simulink model "GRM_Airframe"  (R2018b)
settings: Solver=FixedStepAuto  StartTime=0.0  StopTime=T_sim  FixedStep=0.001  RelTol=1e-3
PreLoadFcn:
  | addpath('init_functions');
  | init_grm;
  | addpath('parameters');
  | para_def_grm;
values from neighbouring files (symbols this model uses):
  act_dmp = 0.6322    [para_def_grm.m]
  act_omega = 59.9250    (= 59.925)    [para_def_grm.m]
  aero = load('aero.mat')    [para_def_grm.m]
  c_be = -6.5e-3    (= -0.0065)    [init_grm.m]
  c_h_geop0 = 0    [init_grm.m]
  c_h_geope = 11e3    (= 11000)    [init_grm.m]
  c_pa0 = 101325    [init_grm.m]
  c_pe = -c_g0/c_be/sgc    (= 5.25587981272)    [init_grm.m]
  c_r0 = 6371000.79    [init_grm.m]
  c_rot = 7.292115e-5    (= 7.292115e-05)    [init_grm.m]
  c_Tmp0 = 288.15    [init_grm.m]
  d_siB_0 = 0    [para_def_grm.m]
  d_siB_max = deg2rad(1200)    [para_def_grm.m]
  d_siB_min = deg2rad(-1200)    [para_def_grm.m]
  dd_siB_max = deg2rad(50000)    [para_def_grm.m]
  dd_siB_min = deg2rad(-50000)    [para_def_grm.m]
  de_JBBB_xx = JBBB_xx_0 - JBBB_xx_e    (= 0)    [para_def_grm.m]
  de_JBBB_yy = JBBB_yy_0 - JBBB_yy_e    (= 0)    [para_def_grm.m]
  de_JBBB_zz = JBBB_zz_0 - JBBB_zz_e    (= 0)    [para_def_grm.m]
  de_mM = m_fuel_lookup(end)    [para_def_grm.m]
  F_prp = [450.52;428.7;423.25;391.61;352.34;304.35;266.17;243.26;216.92 ... (first row only)    [para_def_grm.m]
  flag_I_aero_switch = 1    [init_grm.m]
  flag_I_flat = 1    [init_grm.m]
  flag_I_gravity_switch = 1    [init_grm.m]
  flag_I_rot = 0    [init_grm.m]
  hcr = 1.4    [init_grm.m]
  J0PB_e = TBP*J0PP_e*TBP'    [para_def_grm.m]
  JMMM_0 = TBP*J0PP_0*TBP'    [para_def_grm.m]
  JMMM_e = TBP*J0PP_e*TBP'    [para_def_grm.m]
  lat_0 = 0    [init_grm.m]
  lon_0 = 0    [init_grm.m]
  m0 = mB_0    (= 3.30977)    [para_def_grm.m]
  m_fuel_lookup = [0;0.0573;0.1127;0.1667;0.2186;0.2681;0.3149;0.3588 ... (first row only)    [para_def_grm.m]
  mB_0 = 3.30977    [para_def_grm.m]
  mM_0 = 1.119    [para_def_grm.m]
  mM_e = de_mM    [para_def_grm.m]
  p0PB = [x0PB;y0PB;z0PB]    [para_def_grm.m]
  pBII_0 = TIE_0*pBEE_0    [init_grm.m]
  pMPB = [xMPB;yMPB;zMPB]    [para_def_grm.m]
  pNPB = [0;0;0]    [para_def_grm.m]
  qEG_0 = q12_from_T12(TEG)    [init_grm.m]
  qIB_0 = qumul(qIG_0,qGB_0)    [init_grm.m]
  qIE_0 = q12_from_T12(TIE_0)    [init_grm.m]
  sgc = 287.05287    [init_grm.m]
  siB_0 = 0    [para_def_grm.m]
  siB_max = deg2rad(30)    [para_def_grm.m]
  siB_min = deg2rad(-30)    [para_def_grm.m]
  t_prp1 = [0.04;0.28;0.54;1;1.48;1.99;2.51;3;3.5;3.67;3.82;4]    [para_def_grm.m]
  t_prp2 = t_prp2'    [para_def_grm.m]
  Tr3r4 = [1,1,1,1;1,1,-1,-1;-1,1,1,-1]*0.25    [para_def_grm.m]
  tRRR = 0    [para_def_grm.m]
  unc_act_bl = 0    [para_def_grm.m]
  unc_act_off = 0    [para_def_grm.m]
  unc_act_scale = 1    [para_def_grm.m]
  unc_aero_Cl_scale = 1    [para_def_grm.m]
  unc_aero_Cm_scale = 1    [para_def_grm.m]
  unc_aero_Cn_scale = 1    [para_def_grm.m]
  unc_aero_Cx_scale = 1    [para_def_grm.m]
  unc_aero_Cy_scale = 1    [para_def_grm.m]
  unc_aero_Cz_scale = 1    [para_def_grm.m]
  unc_cg_x = 0    [para_def_grm.m]
  unc_cg_y = 0    [para_def_grm.m]
  unc_cg_z = 0    [para_def_grm.m]
  unc_mB_bl = 0    [para_def_grm.m]
  unc_mB_scale = 1    [para_def_grm.m]
  unc_moi_Jxx = 0    [para_def_grm.m]
  unc_moi_Jyy = 0    [para_def_grm.m]
  unc_moi_Jzz = 0    [para_def_grm.m]
  unc_prp_scale = 1    [para_def_grm.m]
  unc_prp_x = 0    [para_def_grm.m]
  unc_prp_y = 0    [para_def_grm.m]
  unc_prp_z = 0    [para_def_grm.m]
  vBII_0 = vBEE_0 + cross(wIEI_0,pBII_0)    [init_grm.m]
  wBIB_0 = r2_from_r1_trans_q21(wBII_0,qBI_0)    [init_grm.m]
  x0PB = -0.5    [para_def_grm.m]
  xMPB = -0.9    [para_def_grm.m]
  y0PB = 0    [para_def_grm.m]
  yMPB = 0    [para_def_grm.m]
  z0PB = 0    [para_def_grm.m]
  zMPB = 0    [para_def_grm.m]
undefined symbols (not defined in the file or in its folder): c_b_WGS, c_flat, c_grav, c_rsma, d_mB_lookup, t_dmB
libraries: simulink_extras x11, simulink x3
(part 3 of 6)

== system GRM_Airframe/GRM_Airframe/aerodynamics/aerodynamic_via_lookup/calc_aero_for_mom/launch_rail ==
  hBE : Inport
  FBAB_c : Inport  Port=2
  Constant1 : Constant  Value=flag_I_aero_switch
  Constant3 : Constant  Value=0
  Subtract : Sum  Inputs=++-
  Switch : Switch  Criteria=u2 > Threshold  Threshold=0.05
  Vector Concatenate : Concatenate  NumInputs=3
  initial_altitude : Subsystem
  FBAB : Outport
  wires:
  initial_altitude/1(hBE_0) -> Subtract/3
  FBAB_c/1 -> Switch/1
  Vector Concatenate/1 -> Switch/3
  Switch/1 -> FBAB/1  "FBAB"
  Constant3/1 -> Vector Concatenate/3, Vector Concatenate/2, Vector Concatenate/1
  Subtract/1 -> Switch/2
  hBE/1 -> Subtract/1
  Constant1/1 -> Subtract/2

== system GRM_Airframe/GRM_Airframe/aerodynamics/aerodynamic_via_lookup/calc_aero_for_mom/launch_rail1 ==
  hBE : Inport
  MBAB_c : Inport  Port=2
  Constant1 : Constant  Value=flag_I_aero_switch
  Constant3 : Constant  Value=0
  Subtract : Sum  Inputs=++-
  Switch : Switch  Criteria=u2 > Threshold  Threshold=0.05
  Vector Concatenate : Concatenate  NumInputs=3
  initial_altitude : Subsystem
  MBAB : Outport
  wires:
  Constant1/1 -> Subtract/2
  hBE/1 -> Subtract/1
  Subtract/1 -> Switch/2
  Constant3/1 -> Vector Concatenate/1, Vector Concatenate/2, Vector Concatenate/3
  Switch/1 -> MBAB/1  "MBAB"
  Vector Concatenate/1 -> Switch/3
  MBAB_c/1 -> Switch/1
  initial_altitude/1(hBE_0) -> Subtract/3

== system GRM_Airframe/GRM_Airframe/aerodynamics/aerodynamic_via_lookup/calc_derivatives/Cl_derivatives_lookup ==
  aero_pre_lookup : Inport
  Bus Creator1 : BusCreator  Inputs=7
  Bus Selector2 : BusSelector  OutputSignals=k_Mach,f_Mach,k_alB,f_alB,k_beB,f_beB
  Cl_Interpolation : Interpolation_n-D  NumberOfTableDimensions=3  Table=aero.Cl  ExtrapMethod=Clip  DiagnosticForOutOfRangeInput=Warning  InternalRulePriority=Speed
      settings: InputPortMap=u0,u1,u2,u3,u4,u5
  Cl_delta_l_Interpolation : Interpolation_n-D  NumberOfTableDimensions=3  Table=aero.Cl_delta_l  ExtrapMethod=Clip  DiagnosticForOutOfRangeInput=Warning  InternalRulePriority=Speed
      settings: InputPortMap=u0,u1,u2,u3,u4,u5
  Cl_delta_m_Interpolation : Interpolation_n-D  NumberOfTableDimensions=3  Table=aero.Cl_delta_m  ExtrapMethod=Clip  DiagnosticForOutOfRangeInput=Warning  InternalRulePriority=Speed
      settings: InputPortMap=u0,u1,u2,u3,u4,u5
  Cl_delta_n_Interpolation : Interpolation_n-D  NumberOfTableDimensions=3  Table=aero.Cl_delta_n  ExtrapMethod=Clip  DiagnosticForOutOfRangeInput=Warning  InternalRulePriority=Speed
      settings: InputPortMap=u0,u1,u2,u3,u4,u5
  Clp_Interpolation : Interpolation_n-D  NumberOfTableDimensions=3  Table=aero.Clp  ExtrapMethod=Clip  DiagnosticForOutOfRangeInput=Warning  InternalRulePriority=Speed
      settings: InputPortMap=u0,u1,u2,u3,u4,u5
  Clq_Interpolation : Interpolation_n-D  NumberOfTableDimensions=3  Table=aero.Clq  ExtrapMethod=Clip  DiagnosticForOutOfRangeInput=Warning  InternalRulePriority=Speed
      settings: InputPortMap=u0,u1,u2,u3,u4,u5
  Clr_Interpolation : Interpolation_n-D  NumberOfTableDimensions=3  Table=aero.Clr  ExtrapMethod=Clip  DiagnosticForOutOfRangeInput=Warning  InternalRulePriority=Speed
      settings: InputPortMap=u0,u1,u2,u3,u4,u5
  Constant : Constant  Value=unc_aero_Cl_scale
  Product : Product
  Cl_deriv : Outport
  wires:
  Product/1 -> Bus Creator1/1  "Cl"
  Constant/1 -> Product/1
  Bus Creator1/1 -> Cl_deriv/1  "Cl_deriv_bus"
  Clp_Interpolation/1 -> Bus Creator1/2  "Clp"
  Cl_delta_l_Interpolation/1 -> Bus Creator1/5  "Cldl"
  aero_pre_lookup/1 -> Bus Selector2/1
  Cl_Interpolation/1 -> Product/2  "Cl"
  Cl_delta_m_Interpolation/1 -> Bus Creator1/6  "Cldm"
  Clr_Interpolation/1 -> Bus Creator1/4  "Clr"
  Clq_Interpolation/1 -> Bus Creator1/3  "Clq"
  Cl_delta_n_Interpolation/1 -> Bus Creator1/7  "Cldn"
  Bus Selector2/5 -> Cl_Interpolation/5, Clp_Interpolation/5, Clq_Interpolation/5, Clr_Interpolation/5, Cl_delta_l_Interpolation/5, Cl_delta_m_Interpolation/5, Cl_delta_n_Interpolation/5  "<k_beB>"
  Bus Selector2/1 -> Cl_Interpolation/1, Clp_Interpolation/1, Clq_Interpolation/1, Clr_Interpolation/1, Cl_delta_l_Interpolation/1, Cl_delta_m_Interpolation/1, Cl_delta_n_Interpolation/1  "<k_Mach>"
  Bus Selector2/2 -> Cl_Interpolation/2, Clp_Interpolation/2, Clq_Interpolation/2, Clr_Interpolation/2, Cl_delta_l_Interpolation/2, Cl_delta_m_Interpolation/2, Cl_delta_n_Interpolation/2  "<f_Mach>"
  Bus Selector2/3 -> Cl_Interpolation/3, Clp_Interpolation/3, Clq_Interpolation/3, Clr_Interpolation/3, Cl_delta_l_Interpolation/3, Cl_delta_m_Interpolation/3, Cl_delta_n_Interpolation/3  "<k_alB>"
  Bus Selector2/4 -> Cl_Interpolation/4, Clp_Interpolation/4, Clq_Interpolation/4, Clr_Interpolation/4, Cl_delta_l_Interpolation/4, Cl_delta_m_Interpolation/4, Cl_delta_n_Interpolation/4  "<f_alB>"
  Bus Selector2/6 -> Cl_Interpolation/6, Clp_Interpolation/6, Clq_Interpolation/6, Clr_Interpolation/6, Cl_delta_l_Interpolation/6, Cl_delta_m_Interpolation/6, Cl_delta_n_Interpolation/6  "<f_beB>"

== system GRM_Airframe/GRM_Airframe/aerodynamics/aerodynamic_via_lookup/calc_derivatives/Cm_derivatives_lookup ==
  aero_pre_lookup : Inport
  Bus Creator1 : BusCreator  Inputs=7
  Bus Selector2 : BusSelector  OutputSignals=k_Mach,f_Mach,k_alB,f_alB,k_beB,f_beB
  Cm_Interpolation : Interpolation_n-D  NumberOfTableDimensions=3  Table=aero.Cm  ExtrapMethod=Clip  DiagnosticForOutOfRangeInput=Warning  InternalRulePriority=Speed
      settings: InputPortMap=u0,u1,u2,u3,u4,u5
  Cm_delta_l_Interpolation : Interpolation_n-D  NumberOfTableDimensions=3  Table=aero.Cm_delta_l  ExtrapMethod=Clip  DiagnosticForOutOfRangeInput=Warning  InternalRulePriority=Speed
      settings: InputPortMap=u0,u1,u2,u3,u4,u5
  Cm_delta_m_Interpolation : Interpolation_n-D  NumberOfTableDimensions=3  Table=aero.Cm_delta_m  ExtrapMethod=Clip  DiagnosticForOutOfRangeInput=Warning  InternalRulePriority=Speed
      settings: InputPortMap=u0,u1,u2,u3,u4,u5
  Cm_delta_n_Interpolation : Interpolation_n-D  NumberOfTableDimensions=3  Table=aero.Cm_delta_n  ExtrapMethod=Clip  DiagnosticForOutOfRangeInput=Warning  InternalRulePriority=Speed
      settings: InputPortMap=u0,u1,u2,u3,u4,u5
  Cmp_Interpolation : Interpolation_n-D  NumberOfTableDimensions=3  Table=aero.Cmp  ExtrapMethod=Clip  DiagnosticForOutOfRangeInput=Warning  InternalRulePriority=Speed
      settings: InputPortMap=u0,u1,u2,u3,u4,u5
  Cmq_Interpolation : Interpolation_n-D  NumberOfTableDimensions=3  Table=aero.Cmq  ExtrapMethod=Clip  DiagnosticForOutOfRangeInput=Warning  InternalRulePriority=Speed
      settings: InputPortMap=u0,u1,u2,u3,u4,u5
  Cmr_Interpolation : Interpolation_n-D  NumberOfTableDimensions=3  Table=aero.Cmr  ExtrapMethod=Clip  DiagnosticForOutOfRangeInput=Warning  InternalRulePriority=Speed
      settings: InputPortMap=u0,u1,u2,u3,u4,u5
  Constant : Constant  Value=unc_aero_Cm_scale
  Product : Product
  Cm_deriv : Outport
  wires:
  Product/1 -> Bus Creator1/1  "Cm"
  Constant/1 -> Product/1
  Bus Selector2/4 -> Cm_Interpolation/4, Cmp_Interpolation/4, Cmq_Interpolation/4, Cmr_Interpolation/4, Cm_delta_l_Interpolation/4, Cm_delta_m_Interpolation/4, Cm_delta_n_Interpolation/4  "<f_alB>"
  Bus Selector2/3 -> Cm_Interpolation/3, Cmp_Interpolation/3, Cmq_Interpolation/3, Cmr_Interpolation/3, Cm_delta_l_Interpolation/3, Cm_delta_m_Interpolation/3, Cm_delta_n_Interpolation/3  "<k_alB>"
  Bus Selector2/2 -> Cm_Interpolation/2, Cmp_Interpolation/2, Cmq_Interpolation/2, Cmr_Interpolation/2, Cm_delta_l_Interpolation/2, Cm_delta_m_Interpolation/2, Cm_delta_n_Interpolation/2  "<f_Mach>"
  Bus Selector2/1 -> Cm_Interpolation/1, Cmp_Interpolation/1, Cmq_Interpolation/1, Cmr_Interpolation/1, Cm_delta_l_Interpolation/1, Cm_delta_m_Interpolation/1, Cm_delta_n_Interpolation/1  "<k_Mach>"
  Bus Selector2/6 -> Cm_Interpolation/6, Cmp_Interpolation/6, Cmq_Interpolation/6, Cmr_Interpolation/6, Cm_delta_l_Interpolation/6, Cm_delta_m_Interpolation/6, Cm_delta_n_Interpolation/6  "<f_beB>"
  aero_pre_lookup/1 -> Bus Selector2/1
  Cmp_Interpolation/1 -> Bus Creator1/2  "Cmp"
  Cm_delta_l_Interpolation/1 -> Bus Creator1/5  "Cmdl"
  Bus Selector2/5 -> Cm_Interpolation/5, Cmp_Interpolation/5, Cmq_Interpolation/5, Cmr_Interpolation/5, Cm_delta_l_Interpolation/5, Cm_delta_m_Interpolation/5, Cm_delta_n_Interpolation/5  "<k_beB>"
  Cmq_Interpolation/1 -> Bus Creator1/3  "Cmq"
  Cm_Interpolation/1 -> Product/2  "Cm"
  Cm_delta_n_Interpolation/1 -> Bus Creator1/7  "Cmdn"
  Cm_delta_m_Interpolation/1 -> Bus Creator1/6  "Cmdm"
  Cmr_Interpolation/1 -> Bus Creator1/4  "Cmr"
  Bus Creator1/1 -> Cm_deriv/1  "Cm_deriv_bus"

== system GRM_Airframe/GRM_Airframe/aerodynamics/aerodynamic_via_lookup/calc_derivatives/Cn_derivatives_lookup ==
  aero_pre_lookup : Inport
  Bus Creator1 : BusCreator  Inputs=7
  Bus Selector1 : BusSelector  OutputSignals=k_Mach,f_Mach,k_alB,f_alB,k_beB,f_beB
  Cn_Interpolation : Interpolation_n-D  NumberOfTableDimensions=3  Table=aero.Cn  ExtrapMethod=Clip  DiagnosticForOutOfRangeInput=Warning  InternalRulePriority=Speed
      settings: InputPortMap=u0,u1,u2,u3,u4,u5
  Cn_delta_l_Interpolation : Interpolation_n-D  NumberOfTableDimensions=3  Table=aero.Cn_delta_l  ExtrapMethod=Clip  DiagnosticForOutOfRangeInput=Warning  InternalRulePriority=Speed
      settings: InputPortMap=u0,u1,u2,u3,u4,u5
  Cn_delta_m_Interpolation : Interpolation_n-D  NumberOfTableDimensions=3  Table=aero.Cn_delta_m  ExtrapMethod=Clip  DiagnosticForOutOfRangeInput=Warning  InternalRulePriority=Speed
      settings: InputPortMap=u0,u1,u2,u3,u4,u5
  Cn_delta_n_Interpolation : Interpolation_n-D  NumberOfTableDimensions=3  Table=aero.Cn_delta_n  ExtrapMethod=Clip  DiagnosticForOutOfRangeInput=Warning  InternalRulePriority=Speed
      settings: InputPortMap=u0,u1,u2,u3,u4,u5
  Cnp_Interpolation : Interpolation_n-D  NumberOfTableDimensions=3  Table=aero.Cnp  ExtrapMethod=Clip  DiagnosticForOutOfRangeInput=Warning  InternalRulePriority=Speed
      settings: InputPortMap=u0,u1,u2,u3,u4,u5
  Cnq_Interpolation : Interpolation_n-D  NumberOfTableDimensions=3  Table=aero.Cnq  ExtrapMethod=Clip  DiagnosticForOutOfRangeInput=Warning  InternalRulePriority=Speed
      settings: InputPortMap=u0,u1,u2,u3,u4,u5
  Cnr_Interpolation : Interpolation_n-D  NumberOfTableDimensions=3  Table=aero.Cnr  ExtrapMethod=Clip  DiagnosticForOutOfRangeInput=Warning  InternalRulePriority=Speed
      settings: InputPortMap=u0,u1,u2,u3,u4,u5
  Constant : Constant  Value=unc_aero_Cn_scale
  Product : Product
  Cn_deriv : Outport
  wires:
  Product/1 -> Bus Creator1/1  "Cn"
  Constant/1 -> Product/1
  Bus Selector1/6 -> Cn_Interpolation/6, Cnp_Interpolation/6, Cnq_Interpolation/6, Cnr_Interpolation/6, Cn_delta_l_Interpolation/6, Cn_delta_m_Interpolation/6, Cn_delta_n_Interpolation/6  "<f_beB>"
  Cn_delta_l_Interpolation/1 -> Bus Creator1/5  "Cndl"
  Cn_delta_n_Interpolation/1 -> Bus Creator1/7  "Cndn"
  Cn_Interpolation/1 -> Product/2  "Cn"
  Cn_delta_m_Interpolation/1 -> Bus Creator1/6  "Cndm"
  Cnq_Interpolation/1 -> Bus Creator1/3  "Cnq"
  Cnr_Interpolation/1 -> Bus Creator1/4  "Cnr"
  Bus Selector1/5 -> Cn_Interpolation/5, Cnp_Interpolation/5, Cnq_Interpolation/5, Cnr_Interpolation/5, Cn_delta_l_Interpolation/5, Cn_delta_m_Interpolation/5, Cn_delta_n_Interpolation/5  "<k_beB>"
  Bus Creator1/1 -> Cn_deriv/1  "Cn_deriv_bus"
  Cnp_Interpolation/1 -> Bus Creator1/2  "Cnp"
  aero_pre_lookup/1 -> Bus Selector1/1
  Bus Selector1/2 -> Cn_Interpolation/2, Cnp_Interpolation/2, Cnq_Interpolation/2, Cnr_Interpolation/2, Cn_delta_l_Interpolation/2, Cn_delta_m_Interpolation/2, Cn_delta_n_Interpolation/2  "<f_Mach>"
  Bus Selector1/1 -> Cn_Interpolation/1, Cnp_Interpolation/1, Cnq_Interpolation/1, Cnr_Interpolation/1, Cn_delta_l_Interpolation/1, Cn_delta_m_Interpolation/1, Cn_delta_n_Interpolation/1  "<k_Mach>"
  Bus Selector1/4 -> Cn_Interpolation/4, Cnp_Interpolation/4, Cnq_Interpolation/4, Cnr_Interpolation/4, Cn_delta_l_Interpolation/4, Cn_delta_m_Interpolation/4, Cn_delta_n_Interpolation/4  "<f_alB>"
  Bus Selector1/3 -> Cn_Interpolation/3, Cnp_Interpolation/3, Cnq_Interpolation/3, Cnr_Interpolation/3, Cn_delta_l_Interpolation/3, Cn_delta_m_Interpolation/3, Cn_delta_n_Interpolation/3  "<k_alB>"

== system GRM_Airframe/GRM_Airframe/aerodynamics/aerodynamic_via_lookup/calc_derivatives/Cx_derivatives_lookup ==
  delta_t : Inport
  hBE : Inport  Port=2
  aero_pre_lookup : Inport  Port=3
  Bus Creator1 : BusCreator  Inputs=10
  Bus Selector1 : BusSelector  OutputSignals=k_Mach,f_Mach,k_alB,f_alB,k_beB,f_beB
  Constant : Constant  Value=unc_aero_Cx_scale
  Cx_Interpolation : Interpolation_n-D  NumberOfTableDimensions=3  Table=aero.Cx  ExtrapMethod=Clip  InternalRulePriority=Speed
      settings: InputPortMap=u0,u1,u2,u3,u4,u5
  Cx_alt_Interpolation : Interpolation_n-D  NumberOfTableDimensions=3  Table=aero.Cx_alt  ExtrapMethod=Clip  InternalRulePriority=Speed
      settings: InputPortMap=u0,u1,u2,u3,u4,u5
  Cx_base_Interpolation : Interpolation_n-D  NumberOfTableDimensions=3  Table=aero.Cx_base  ExtrapMethod=Clip  InternalRulePriority=Speed
      settings: InputPortMap=u0,u1,u2,u3,u4,u5
  Cx_delta_l_Interpolation : Interpolation_n-D  NumberOfTableDimensions=3  Table=aero.Cx_delta_l  ExtrapMethod=Clip  InternalRulePriority=Speed
      settings: InputPortMap=u0,u1,u2,u3,u4,u5
  Cx_delta_m_Interpolation : Interpolation_n-D  NumberOfTableDimensions=3  Table=aero.Cx_delta_m  ExtrapMethod=Clip  InternalRulePriority=Speed
      settings: InputPortMap=u0,u1,u2,u3,u4,u5
  Cx_delta_n_Interpolation : Interpolation_n-D  NumberOfTableDimensions=3  Table=aero.Cx_delta_n  ExtrapMethod=Clip  InternalRulePriority=Speed
      settings: InputPortMap=u0,u1,u2,u3,u4,u5
  Cx_delta_t_Interpolation : Interpolation_n-D  NumberOfTableDimensions=3  Table=aero.Cx_delta_t  ExtrapMethod=Clip  InternalRulePriority=Speed
      settings: InputPortMap=u0,u1,u2,u3,u4,u5
  Cxp_Interpolation : Interpolation_n-D  NumberOfTableDimensions=3  Table=aero.Cxp  ExtrapMethod=Clip  InternalRulePriority=Speed
      settings: InputPortMap=u0,u1,u2,u3,u4,u5
  Cxq_Interpolation : Interpolation_n-D  NumberOfTableDimensions=3  Table=aero.Cxq  ExtrapMethod=Clip  InternalRulePriority=Speed
      settings: InputPortMap=u0,u1,u2,u3,u4,u5
  Cxr_Interpolation : Interpolation_n-D  NumberOfTableDimensions=3  Table=aero.Cxr  ExtrapMethod=Clip  InternalRulePriority=Speed
      settings: InputPortMap=u0,u1,u2,u3,u4,u5
  Prelookup_altitude : PreLookup  BreakpointsData=aero.hoehe
  Prelookup_delta_t : PreLookup  BreakpointsData=aero.delta_t
  Product : Product
  Cx_deriv : Outport
  wires:
  Constant/1 -> Product/1
  Product/1 -> Bus Creator1/1  "Cx"
  Cx_delta_n_Interpolation/1 -> Bus Creator1/7  "Cxdn"
  Cx_delta_m_Interpolation/1 -> Bus Creator1/6  "Cxdm"
  Cx_delta_l_Interpolation/1 -> Bus Creator1/5  "Cxdl"
  delta_t/1 -> Prelookup_delta_t/1
  Bus Creator1/1 -> Cx_deriv/1  "Cx_deriv_bus"
  Prelookup_altitude/2 -> Cx_alt_Interpolation/6
  Prelookup_altitude/1 -> Cx_alt_Interpolation/5
  hBE/1 -> Prelookup_altitude/1
  aero_pre_lookup/1 -> Bus Selector1/1
  Prelookup_delta_t/1 -> Cx_delta_t_Interpolation/5
  Bus Selector1/1 -> Cx_Interpolation/1, Cxp_Interpolation/1, Cxq_Interpolation/1, Cxr_Interpolation/1, Cx_delta_l_Interpolation/1, Cx_alt_Interpolation/1, Cx_delta_t_Interpolation/1, Cx_base_Interpolation/1, Cx_delta_n_Interpolation/1, Cx_delta_m_Interpolation/1  "<k_Mach>"
  Bus Selector1/2 -> Cx_Interpolation/2, Cxp_Interpolation/2, Cxq_Interpolation/2, Cxr_Interpolation/2, Cx_delta_l_Interpolation/2, Cx_base_Interpolation/2, Cx_alt_Interpolation/2, Cx_delta_t_Interpolation/2, Cx_delta_n_Interpolation/2, Cx_delta_m_Interpolation/2  "<f_Mach>"
  Prelookup_delta_t/2 -> Cx_delta_t_Interpolation/6
  Bus Selector1/3 -> Cx_Interpolation/3, Cxp_Interpolation/3, Cxq_Interpolation/3, Cxr_Interpolation/3, Cx_delta_l_Interpolation/3, Cx_alt_Interpolation/3, Cx_delta_t_Interpolation/3, Cx_base_Interpolation/3, Cx_delta_n_Interpolation/3, Cx_delta_m_Interpolation/3  "<k_alB>"
  Bus Selector1/6 -> Cxp_Interpolation/6, Cxq_Interpolation/6, Cxr_Interpolation/6, Cx_delta_l_Interpolation/6, Cx_base_Interpolation/6, Cx_delta_n_Interpolation/6, Cx_delta_m_Interpolation/6, Cx_Interpolation/6  "<f_beB>"
  Bus Selector1/4 -> Cx_Interpolation/4, Cxp_Interpolation/4, Cxq_Interpolation/4, Cxr_Interpolation/4, Cx_delta_l_Interpolation/4, Cx_alt_Interpolation/4, Cx_delta_t_Interpolation/4, Cx_base_Interpolation/4, Cx_delta_n_Interpolation/4, Cx_delta_m_Interpolation/4  "<f_alB>"
  Cxp_Interpolation/1 -> Bus Creator1/2  "Cxp"
  Cx_delta_t_Interpolation/1 -> Bus Creator1/10  "Cx_alB_t"
  Cxr_Interpolation/1 -> Bus Creator1/4  "Cxr"
  Cxq_Interpolation/1 -> Bus Creator1/3  "Cxq"
  Cx_base_Interpolation/1 -> Bus Creator1/8  "Cx_base"
  Cx_Interpolation/1 -> Product/2  "Cx"
  Cx_alt_Interpolation/1 -> Bus Creator1/9  "Cx_alt"
  Bus Selector1/5 -> Cxp_Interpolation/5, Cxq_Interpolation/5, Cxr_Interpolation/5, Cx_delta_l_Interpolation/5, Cx_base_Interpolation/5, Cx_delta_n_Interpolation/5, Cx_delta_m_Interpolation/5, Cx_Interpolation/5  "<k_beB>"

== system GRM_Airframe/GRM_Airframe/aerodynamics/aerodynamic_via_lookup/calc_derivatives/Cy_derivatives_lookup ==
  aero_pre_lookup : Inport
  Bus Creator1 : BusCreator  Inputs=7
  Bus Selector1 : BusSelector  OutputSignals=k_Mach,f_Mach,k_alB,f_alB,k_beB,f_beB
  Constant : Constant  Value=unc_aero_Cy_scale
  Cy_Interpolation : Interpolation_n-D  NumberOfTableDimensions=3  Table=aero.Cy  ExtrapMethod=Clip  InternalRulePriority=Speed
      settings: InputPortMap=u0,u1,u2,u3,u4,u5
  Cy_delta_l_Interpolation : Interpolation_n-D  NumberOfTableDimensions=3  Table=aero.Cy_delta_l  ExtrapMethod=Clip  InternalRulePriority=Speed
      settings: InputPortMap=u0,u1,u2,u3,u4,u5
  Cy_delta_m_Interpolation : Interpolation_n-D  NumberOfTableDimensions=3  Table=aero.Cy_delta_m  ExtrapMethod=Clip  InternalRulePriority=Speed
      settings: InputPortMap=u0,u1,u2,u3,u4,u5
  Cy_delta_n_Interpolation : Interpolation_n-D  NumberOfTableDimensions=3  Table=aero.Cy_delta_n  ExtrapMethod=Clip  InternalRulePriority=Speed
      settings: InputPortMap=u0,u1,u2,u3,u4,u5
  Cyp_Interpolation : Interpolation_n-D  NumberOfTableDimensions=3  Table=aero.Cyp  ExtrapMethod=Clip  InternalRulePriority=Speed
      settings: InputPortMap=u0,u1,u2,u3,u4,u5
  Cyq_Interpolation : Interpolation_n-D  NumberOfTableDimensions=3  Table=aero.Cyq  ExtrapMethod=Clip  InternalRulePriority=Speed
      settings: InputPortMap=u0,u1,u2,u3,u4,u5
  Cyr_Interpolation : Interpolation_n-D  NumberOfTableDimensions=3  Table=aero.Cyr  ExtrapMethod=Clip  InternalRulePriority=Speed
      settings: InputPortMap=u0,u1,u2,u3,u4,u5
  Product : Product
  Cy_deriv : Outport
  wires:
  Product/1 -> Bus Creator1/1  "Cy"
  Constant/1 -> Product/1
  Cyq_Interpolation/1 -> Bus Creator1/3  "Cyq"
  Cyr_Interpolation/1 -> Bus Creator1/4  "Cyr"
  Bus Creator1/1 -> Cy_deriv/1  "Cy_deriv_bus"
  Cy_delta_m_Interpolation/1 -> Bus Creator1/6  "Cydm"
  Cy_delta_l_Interpolation/1 -> Bus Creator1/5  "Cydl"
  Cyp_Interpolation/1 -> Bus Creator1/2  "Cyp"
  aero_pre_lookup/1 -> Bus Selector1/1
  Bus Selector1/2 -> Cy_Interpolation/2, Cyp_Interpolation/2, Cyq_Interpolation/2, Cyr_Interpolation/2, Cy_delta_l_Interpolation/2, Cy_delta_m_Interpolation/2, Cy_delta_n_Interpolation/2  "<f_Mach>"
  Bus Selector1/1 -> Cy_Interpolation/1, Cyp_Interpolation/1, Cyq_Interpolation/1, Cyr_Interpolation/1, Cy_delta_l_Interpolation/1, Cy_delta_m_Interpolation/1, Cy_delta_n_Interpolation/1  "<k_Mach>"
  Bus Selector1/3 -> Cy_Interpolation/3, Cyp_Interpolation/3, Cyq_Interpolation/3, Cyr_Interpolation/3, Cy_delta_l_Interpolation/3, Cy_delta_m_Interpolation/3, Cy_delta_n_Interpolation/3  "<k_alB>"
  Bus Selector1/4 -> Cy_Interpolation/4, Cyp_Interpolation/4, Cyq_Interpolation/4, Cyr_Interpolation/4, Cy_delta_l_Interpolation/4, Cy_delta_m_Interpolation/4, Cy_delta_n_Interpolation/4  "<f_alB>"
  Bus Selector1/6 -> Cy_Interpolation/6, Cyp_Interpolation/6, Cyq_Interpolation/6, Cyr_Interpolation/6, Cy_delta_l_Interpolation/6, Cy_delta_m_Interpolation/6, Cy_delta_n_Interpolation/6  "<f_beB>"
  Bus Selector1/5 -> Cy_Interpolation/5, Cyp_Interpolation/5, Cyq_Interpolation/5, Cyr_Interpolation/5, Cy_delta_l_Interpolation/5, Cy_delta_m_Interpolation/5, Cy_delta_n_Interpolation/5  "<k_beB>"
  Cy_delta_n_Interpolation/1 -> Bus Creator1/7  "Cydn"
  Cy_Interpolation/1 -> Product/2  "Cy"

== system GRM_Airframe/GRM_Airframe/aerodynamics/aerodynamic_via_lookup/calc_derivatives/Cz_derivatives_lookup ==
  aero_pre_lookup : Inport
  Bus Creator1 : BusCreator  Inputs=7
  Bus Selector2 : BusSelector  OutputSignals=k_Mach,f_Mach,k_alB,f_alB,k_beB,f_beB
  Constant : Constant  Value=unc_aero_Cz_scale
  Cz_Interpolation : Interpolation_n-D  NumberOfTableDimensions=3  Table=aero.Cz  ExtrapMethod=Clip  DiagnosticForOutOfRangeInput=Warning  InternalRulePriority=Speed
      settings: InputPortMap=u0,u1,u2,u3,u4,u5
  Cz_delta_l_Interpolation : Interpolation_n-D  NumberOfTableDimensions=3  Table=aero.Cz_delta_l  ExtrapMethod=Clip  DiagnosticForOutOfRangeInput=Warning  InternalRulePriority=Speed
      settings: InputPortMap=u0,u1,u2,u3,u4,u5
  Cz_delta_m_Interpolation : Interpolation_n-D  NumberOfTableDimensions=3  Table=aero.Cz_delta_m  ExtrapMethod=Clip  DiagnosticForOutOfRangeInput=Warning  InternalRulePriority=Speed
      settings: InputPortMap=u0,u1,u2,u3,u4,u5
  Cz_delta_n_Interpolation : Interpolation_n-D  NumberOfTableDimensions=3  Table=aero.Cz_delta_n  ExtrapMethod=Clip  DiagnosticForOutOfRangeInput=Warning  InternalRulePriority=Speed
      settings: InputPortMap=u0,u1,u2,u3,u4,u5
  Czp_Interpolation : Interpolation_n-D  NumberOfTableDimensions=3  Table=aero.Czp  ExtrapMethod=Clip  DiagnosticForOutOfRangeInput=Warning  InternalRulePriority=Speed
      settings: InputPortMap=u0,u1,u2,u3,u4,u5
  Czq_Interpolation : Interpolation_n-D  NumberOfTableDimensions=3  Table=aero.Czq  ExtrapMethod=Clip  DiagnosticForOutOfRangeInput=Warning  InternalRulePriority=Speed
      settings: InputPortMap=u0,u1,u2,u3,u4,u5
  Czr_Interpolation : Interpolation_n-D  NumberOfTableDimensions=3  Table=aero.Czr  ExtrapMethod=Clip  DiagnosticForOutOfRangeInput=Warning  InternalRulePriority=Speed
      settings: InputPortMap=u0,u1,u2,u3,u4,u5
  Product : Product
  Cz_deriv : Outport
  wires:
  Product/1 -> Bus Creator1/1  "Cz"
  Constant/1 -> Product/1
  Czr_Interpolation/1 -> Bus Creator1/4  "Czr"
  Czp_Interpolation/1 -> Bus Creator1/2  "Czp"
  aero_pre_lookup/1 -> Bus Selector2/1
  Czq_Interpolation/1 -> Bus Creator1/3  "Czq"
  Bus Creator1/1 -> Cz_deriv/1  "Cz_deriv_bus"
  Cz_delta_l_Interpolation/1 -> Bus Creator1/5  "Czdl"
  Cz_delta_n_Interpolation/1 -> Bus Creator1/7  "Czdn"
  Bus Selector2/3 -> Cz_Interpolation/3, Czp_Interpolation/3, Czq_Interpolation/3, Czr_Interpolation/3, Cz_delta_l_Interpolation/3, Cz_delta_m_Interpolation/3, Cz_delta_n_Interpolation/3  "<k_alB>"
  Bus Selector2/6 -> Cz_Interpolation/6, Czp_Interpolation/6, Czq_Interpolation/6, Czr_Interpolation/6, Cz_delta_l_Interpolation/6, Cz_delta_m_Interpolation/6, Cz_delta_n_Interpolation/6  "<f_beB>"
  Cz_delta_m_Interpolation/1 -> Bus Creator1/6  "Czdm"
  Cz_Interpolation/1 -> Product/2  "Cz"
  Bus Selector2/5 -> Cz_Interpolation/5, Czp_Interpolation/5, Czq_Interpolation/5, Czr_Interpolation/5, Cz_delta_l_Interpolation/5, Cz_delta_m_Interpolation/5, Cz_delta_n_Interpolation/5  "<k_beB>"
  Bus Selector2/1 -> Cz_Interpolation/1, Czp_Interpolation/1, Czq_Interpolation/1, Czr_Interpolation/1, Cz_delta_l_Interpolation/1, Cz_delta_m_Interpolation/1, Cz_delta_n_Interpolation/1  "<k_Mach>"
  Bus Selector2/2 -> Cz_Interpolation/2, Czp_Interpolation/2, Czq_Interpolation/2, Czr_Interpolation/2, Cz_delta_l_Interpolation/2, Cz_delta_m_Interpolation/2, Cz_delta_n_Interpolation/2  "<f_Mach>"
  Bus Selector2/4 -> Cz_Interpolation/4, Czp_Interpolation/4, Czq_Interpolation/4, Czr_Interpolation/4, Cz_delta_l_Interpolation/4, Cz_delta_m_Interpolation/4, Cz_delta_n_Interpolation/4  "<f_alB>"

== system GRM_Airframe/GRM_Airframe/aerodynamics/aerodynamic_via_lookup/calc_derivatives/aerodynamics_pre_lookup ==
  alB : Inport
  beB : Inport  Port=2
  Ma : Inport  Port=3
  Bus Creator1 : BusCreator  Inputs=6
  Prelookup_Mach : PreLookup  BreakpointsData=aero.Ma
  Prelookup_alB : PreLookup  BreakpointsData=aero.alpha
  Prelookup_beB : PreLookup  BreakpointsData=aero.beta
  aero_pre_lookup : Outport
  wires:
  beB/1 -> Prelookup_beB/1
  alB/1 -> Prelookup_alB/1
  Prelookup_beB/2 -> Bus Creator1/6  "f_beB"
  Prelookup_beB/1 -> Bus Creator1/5  "k_beB"
  Prelookup_Mach/1 -> Bus Creator1/1  "k_Mach"
  Prelookup_Mach/2 -> Bus Creator1/2  "f_Mach"
  Ma/1 -> Prelookup_Mach/1
  Prelookup_alB/2 -> Bus Creator1/4  "f_alB"
  Prelookup_alB/1 -> Bus Creator1/3  "k_alB"
  Bus Creator1/1 -> aero_pre_lookup/1  "aero_pre_lookup_bus"

== system GRM_Airframe/GRM_Airframe/aerodynamics/aerodynamic_via_lookup/calc_derivatives/calc_total_deflection_angle ==
  etB_deg : Inport
  zeB_deg : Inport  Port=2
  alB : Inport  Port=3
  beB : Inport  Port=4
  Abs : Abs
  Abs1 : Abs
  Abs2 : Abs
  Add : Sum
  Constant3 : Constant  Value=2
  Degrees to Radians : simulink_extras/Transformations/Degrees to Radians
  Degrees to Radians1 : simulink_extras/Transformations/Degrees to Radians
  Divide2 : Product  Inputs=**/
  Product1 : Product
  Product6 : Product
  Product7 : Product
  Radians to Degrees1 : simulink_extras/Transformations/Radians to Degrees
  Saturation : Saturate  UpperLimit=inf  LowerLimit=100*eps
      settings: AttributesFormatString=|
      | %<UpperLimit>
      | %<LowerLimit>
  Sqrt : Sqrt  SaturateOnIntegerOverflow=on
  Trigonometric Function : Trigonometry  Operator=acos
  Trigonometric Function1 : Trigonometry  Operator=cos
  Trigonometric Function2 : Trigonometry  Operator=cos
  delta_t : Outport
  wires:
  Radians to Degrees1/1 -> Saturation/1  "alB_t_deg"
  Trigonometric Function/1 -> Radians to Degrees1/1  "alB_t"
  Degrees to Radians1/1 -> Trigonometric Function2/1
  Degrees to Radians/1 -> Trigonometric Function1/1
  Abs2/1 -> delta_t/1  "delta_t"
  alB/1 -> Degrees to Radians/1, Abs/1
  Product1/1 -> Trigonometric Function/1
  Sqrt/1 -> Divide2/2
  Product7/1 -> Add/2
  beB/1 -> Degrees to Radians1/1, Abs1/1
  Add/1 -> Divide2/1
  Trigonometric Function1/1 -> Product1/1
  Constant3/1 -> Sqrt/1
  zeB_deg/1 -> Product7/2
  Abs/1 -> Product6/1
  etB_deg/1 -> Product6/2
  Trigonometric Function2/1 -> Product1/2
  Divide2/1 -> Abs2/1
  Abs1/1 -> Product7/1
  Saturation/1 -> Divide2/3
  Product6/1 -> Add/1

== system GRM_Airframe/GRM_Airframe/environment/WGS84_Gravitation/WGS84_2_ECEF/WGS84 Transformation Parameter  ==
  phi : Inport
  Add2 : Sum  Inputs=+-
  Divide : Product  Inputs=**
  Divide1 : Product  Inputs=**
  Divide2 : Product  Inputs=**
  Divide3 : Product  Inputs=/*
  Sqrt : Sqrt  SaturateOnIntegerOverflow=on
  Subsystem : Subsystem
  Trigonometric Function : Trigonometry
  "WGS84 Semi-major Axis, [m]" : Constant  Value=c_rsma
  "WGS84 Semi-minor Axis, [m]" : Constant  Value=c_b_WGS
  a3 : Constant
  N : Outport
  e : Outport  Port=2
  wires:
  phi/1 -> Trigonometric Function/1
  Add2/1 -> Sqrt/1
  Subsystem/1(e) -> Divide/1, Divide/2, e/1
  Divide/1 -> Divide2/2  "e^2"
  Trigonometric Function/1 -> Divide1/1, Divide1/2
  Divide2/1 -> Add2/2
  a3/1 -> Add2/1
  Sqrt/1 -> Divide3/1
  Divide3/1 -> N/1  "N"
  Divide1/1 -> Divide2/1  "sin(phi)^2"
  "WGS84 Semi-major Axis, [m]"/1 -> Divide3/2, Subsystem/2(a)  "c_rsma"
  "WGS84 Semi-minor Axis, [m]"/1 -> Subsystem/1(b)  "c_b_WGS"

== system GRM_Airframe/GRM_Airframe/environment/atmosphere_static_ISO_2533/tmp_and_pressure_ISO_2533/static_Temperature ==
  Tmp_ref : Inport
  h_geop : Inport  Port=2
  h_geop_ref : Inport  Port=3
  Add : Sum
  Product : Product
  Subtract : Sum  Inputs=+-
  Tmp_gradient_tropo : Constant  Value=c_be
  Tmp : Outport
  wires:
  h_geop_ref/1 -> Subtract/2
  h_geop/1 -> Subtract/1
  Tmp_ref/1 -> Add/1
  Add/1 -> Tmp/1  "Tmp"
  Product/1 -> Add/2
  Tmp_gradient_tropo/1 -> Product/1
  Subtract/1 -> Product/2

== system GRM_Airframe/GRM_Airframe/environment/atmosphere_static_ISO_2533/tmp_and_pressure_ISO_2533/static_pressure ==
  h_geop_ref : Inport
  h_geop : Inport  Port=2
  Tmp_ref : Inport  Port=3
  pa_ref : Inport  Port=4
  Add : Sum
  Constant1 : Constant
  Divide : Product  Inputs=*/*
  Math Function : Math  Operator=pow  SaturateOnIntegerOverflow=on
  Product : Product
  Subtract : Sum  Inputs=-+
  Tmp_gradient_tropo : Constant  Value=c_be
  pressure_exponent : Constant  Value=c_pe
  pa : Outport
  wires:
  Tmp_gradient_tropo/1 -> Divide/3
  Product/1 -> pa/1  "pa"
  Constant1/1 -> Add/1
  Subtract/1 -> Divide/1
  Math Function/1 -> Product/1
  pa_ref/1 -> Product/2
  Add/1 -> Math Function/1
  Tmp_ref/1 -> Divide/2
  h_geop_ref/1 -> Subtract/1
  Divide/1 -> Add/2
  h_geop/1 -> Subtract/2
  pressure_exponent/1 -> Math Function/2

== system GRM_Airframe/GRM_Airframe/gravity/launch_rail/initial_altitude/trafo_E_to_geodetic ==
  note: Inputs [size]:
      |
      | position_E [3]
  note: Outputs [size]:
      |
      | geodetic longitude [1]
      | geodetic latitude [1]
      | geodetic altitude [1]
  pBEE : Inport
  Geodetic_altitude : Subsystem
  Geodetic_latitude : Subsystem
  Selector1 : Selector  IndexMode=Zero-based  InputPortWidth=3  IndexOptions=Index vector (dialog)  Indices=1  OutputSizes=1
  Selector2 : Selector  IndexMode=Zero-based  InputPortWidth=3  IndexOptions=Index vector (dialog)  Indices=0  OutputSizes=1
  Trigonometric Function1 : Trigonometry  Operator=atan2
  c_flat : Constant  Value=c_flat
  c_rsma : Constant  Value=c_rsma
  lon : Outport
  lat : Outport  Port=2
  alt : Outport  Port=3
  wires:
  pBEE/1 -> Geodetic_altitude/1(pBEE), Geodetic_latitude/1(pBEE), Selector2/1, Selector1/1  "pBEE"
  Trigonometric Function1/1 -> lon/1  "lon"
  Geodetic_altitude/1(alt) -> alt/1
  Geodetic_latitude/1(lat) -> lat/1, Geodetic_altitude/4(lat)
  Selector2/1 -> Trigonometric Function1/2  "pBEE_x"
  Selector1/1 -> Trigonometric Function1/1  "pBEE_y"
  c_rsma/1 -> Geodetic_altitude/2(c_rsma), Geodetic_latitude/2(c_rsma)  "c_rsma"
  c_flat/1 -> Geodetic_latitude/3(c_flat), Geodetic_altitude/3(c_flat)  "c_flat"

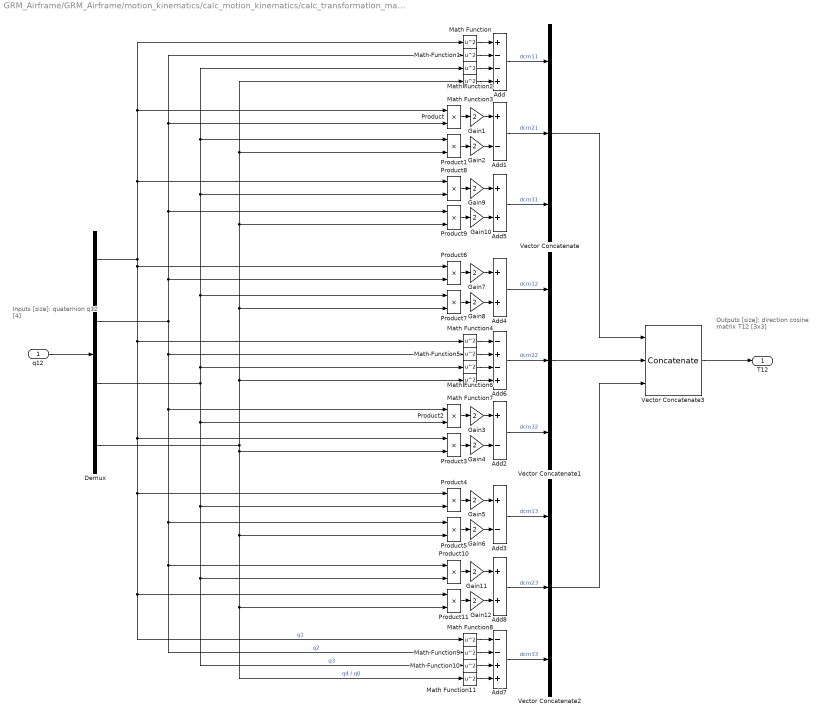
== system GRM_Airframe/GRM_Airframe/motion_kinematics/calc_motion_kinematics/calc_transformation_matrix/T12_from_q1 ==
  note: Outputs [size]:
      |
      | direction cosine matrix T12 [3x3]
  note: Inputs [size]:
      |
      | quaternion q12 [4]
  q12 : Inport  PortDimensions=4
  Add : Sum  Inputs=+--+
  Add1 : Sum  Inputs=+-
  Add2 : Sum  Inputs=+-
  Add3 : Sum  Inputs=+-
  Add4 : Sum
  Add5 : Sum
  Add6 : Sum  Inputs=-+-+
  Add7 : Sum  Inputs=--++
  Add8 : Sum
  Demux : Demux
  Gain{1..12} (12 alike) : Gain  Gain=2
  Math Function{,1..11} (12 alike) : Math  Operator=square  SaturateOnIntegerOverflow=on
  Product{,1..11} (12 alike) : Product
  Vector Concatenate : Concatenate  NumInputs=3
  Vector Concatenate1 : Concatenate  NumInputs=3
  Vector Concatenate2 : Concatenate  NumInputs=3
  Vector Concatenate3 : Concatenate  NumInputs=3  Mode=Multidimensional array  ConcatenateDimension=2
  T12 : Outport  PortDimensions=[3 3]
  wires:
  q12/1 -> Demux/1
  Demux/1 -> Product8/1, Product/1, Math Function/1, Product3/1, Product4/1, Product11/1, Math Function8/1, Math Function4/1, Product6/1  "q1"
  Demux/2 -> Product2/1, Product5/1, Product10/1, Math Function9/1, Math Function5/1, Product6/2, Product9/1, Product/2, Math Function1/1  "q2"
  Demux/3 -> Product2/2, Product4/2, Math Function10/1, Product10/2, Math Function6/1, Product7/1, Product8/2, Product1/1, Math Function2/1  "q3"
  Demux/4 -> Math Function7/1, Product7/2, Product9/2, Product1/2, Math Function3/1, Product5/2, Math Function11/1, Product11/2, Product3/2  "q4 / q0"
  Vector Concatenate3/1 -> T12/1
  Vector Concatenate/1 -> Vector Concatenate3/1
  Vector Concatenate2/1 -> Vector Concatenate3/3
  Vector Concatenate1/1 -> Vector Concatenate3/2
  Add/1 -> Vector Concatenate/1  "dcm11"
  Add1/1 -> Vector Concatenate/2  "dcm21"
  Add5/1 -> Vector Concatenate/3  "dcm31"
  Add4/1 -> Vector Concatenate1/1  "dcm12"
  Add6/1 -> Vector Concatenate1/2  "dcm22"
  Add2/1 -> Vector Concatenate1/3  "dcm32"
  Add3/1 -> Vector Concatenate2/1  "dcm13"
  Add8/1 -> Vector Concatenate2/2  "dcm23"
  Add7/1 -> Vector Concatenate2/3  "dcm33"
  Math Function/1 -> Add/1
  Math Function1/1 -> Add/2
  Math Function2/1 -> Add/3
  Math Function3/1 -> Add/4
  Product/1 -> Gain1/1
  Product1/1 -> Gain2/1
  Gain1/1 -> Add1/1
  Gain2/1 -> Add1/2
  Gain4/1 -> Add2/2
  Gain3/1 -> Add2/1
  Product3/1 -> Gain4/1
  Product2/1 -> Gain3/1
  Gain6/1 -> Add3/2
  Gain5/1 -> Add3/1
  Product5/1 -> Gain6/1
  Product4/1 -> Gain5/1
  Gain8/1 -> Add4/2
  Gain7/1 -> Add4/1
  Product7/1 -> Gain8/1
  Product6/1 -> Gain7/1
  Gain10/1 -> Add5/2
  Gain9/1 -> Add5/1
  Product9/1 -> Gain10/1
  Product8/1 -> Gain9/1
  Math Function6/1 -> Add6/3
  Math Function7/1 -> Add6/4
  Math Function5/1 -> Add6/2
  Math Function4/1 -> Add6/1
  Math Function10/1 -> Add7/3
  Math Function11/1 -> Add7/4
  Math Function9/1 -> Add7/2
  Math Function8/1 -> Add7/1
  Gain12/1 -> Add8/2
  Gain11/1 -> Add8/1
  Product11/1 -> Gain12/1
  Product10/1 -> Gain11/1

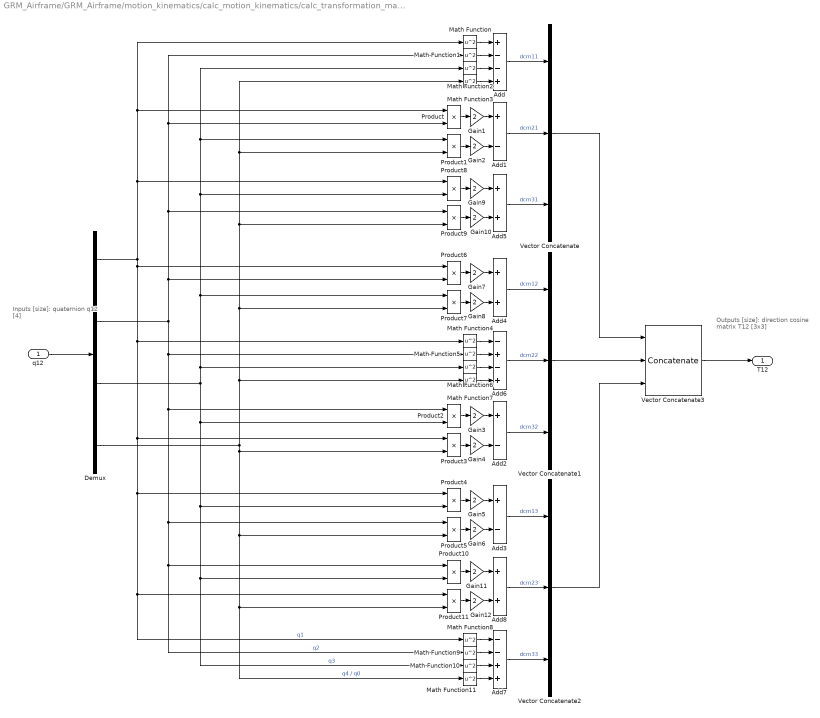
== system GRM_Airframe/GRM_Airframe/motion_kinematics/calc_motion_kinematics/calc_transformation_matrix/T12_from_q12 ==
  note: Outputs [size]:
      |
      | direction cosine matrix T12 [3x3]
  note: Inputs [size]:
      |
      | quaternion q12 [4]
  q12 : Inport  PortDimensions=4
  Add : Sum  Inputs=+--+
  Add1 : Sum  Inputs=+-
  Add2 : Sum  Inputs=+-
  Add3 : Sum  Inputs=+-
  Add4 : Sum
  Add5 : Sum
  Add6 : Sum  Inputs=-+-+
  Add7 : Sum  Inputs=--++
  Add8 : Sum
  Demux : Demux
  Gain{1..12} (12 alike) : Gain  Gain=2
  Math Function{,1..11} (12 alike) : Math  Operator=square  SaturateOnIntegerOverflow=on
  Product{,1..11} (12 alike) : Product
  Vector Concatenate : Concatenate  NumInputs=3
  Vector Concatenate1 : Concatenate  NumInputs=3
  Vector Concatenate2 : Concatenate  NumInputs=3
  Vector Concatenate3 : Concatenate  NumInputs=3  Mode=Multidimensional array  ConcatenateDimension=2
  T12 : Outport  PortDimensions=[3 3]
  wires:
  q12/1 -> Demux/1
  Demux/1 -> Product8/1, Product/1, Math Function/1, Product3/1, Product4/1, Product11/1, Math Function8/1, Math Function4/1, Product6/1  "q1"
  Demux/2 -> Product2/1, Product5/1, Product10/1, Math Function9/1, Math Function5/1, Product6/2, Product9/1, Product/2, Math Function1/1  "q2"
  Demux/3 -> Product2/2, Product4/2, Math Function10/1, Product10/2, Math Function6/1, Product7/1, Product8/2, Product1/1, Math Function2/1  "q3"
  Demux/4 -> Math Function7/1, Product7/2, Product9/2, Product1/2, Math Function3/1, Product5/2, Math Function11/1, Product11/2, Product3/2  "q4 / q0"
  Vector Concatenate3/1 -> T12/1
  Vector Concatenate/1 -> Vector Concatenate3/1
  Vector Concatenate2/1 -> Vector Concatenate3/3
  Vector Concatenate1/1 -> Vector Concatenate3/2
  Add/1 -> Vector Concatenate/1  "dcm11"
  Add1/1 -> Vector Concatenate/2  "dcm21"
  Add5/1 -> Vector Concatenate/3  "dcm31"
  Add4/1 -> Vector Concatenate1/1  "dcm12"
  Add6/1 -> Vector Concatenate1/2  "dcm22"
  Add2/1 -> Vector Concatenate1/3  "dcm32"
  Add3/1 -> Vector Concatenate2/1  "dcm13"
  Add8/1 -> Vector Concatenate2/2  "dcm23"
  Add7/1 -> Vector Concatenate2/3  "dcm33"
  Math Function/1 -> Add/1
  Math Function1/1 -> Add/2
  Math Function2/1 -> Add/3
  Math Function3/1 -> Add/4
  Product/1 -> Gain1/1
  Product1/1 -> Gain2/1
  Gain1/1 -> Add1/1
  Gain2/1 -> Add1/2
  Gain4/1 -> Add2/2
  Gain3/1 -> Add2/1
  Product3/1 -> Gain4/1
  Product2/1 -> Gain3/1
  Gain6/1 -> Add3/2
  Gain5/1 -> Add3/1
  Product5/1 -> Gain6/1
  Product4/1 -> Gain5/1
  Gain8/1 -> Add4/2
  Gain7/1 -> Add4/1
  Product7/1 -> Gain8/1
  Product6/1 -> Gain7/1
  Gain10/1 -> Add5/2
  Gain9/1 -> Add5/1
  Product9/1 -> Gain10/1
  Product8/1 -> Gain9/1
  Math Function6/1 -> Add6/3
  Math Function7/1 -> Add6/4
  Math Function5/1 -> Add6/2
  Math Function4/1 -> Add6/1
  Math Function10/1 -> Add7/3
  Math Function11/1 -> Add7/4
  Math Function9/1 -> Add7/2
  Math Function8/1 -> Add7/1
  Gain12/1 -> Add8/2
  Gain11/1 -> Add8/1
  Product11/1 -> Gain12/1
  Product10/1 -> Gain11/1

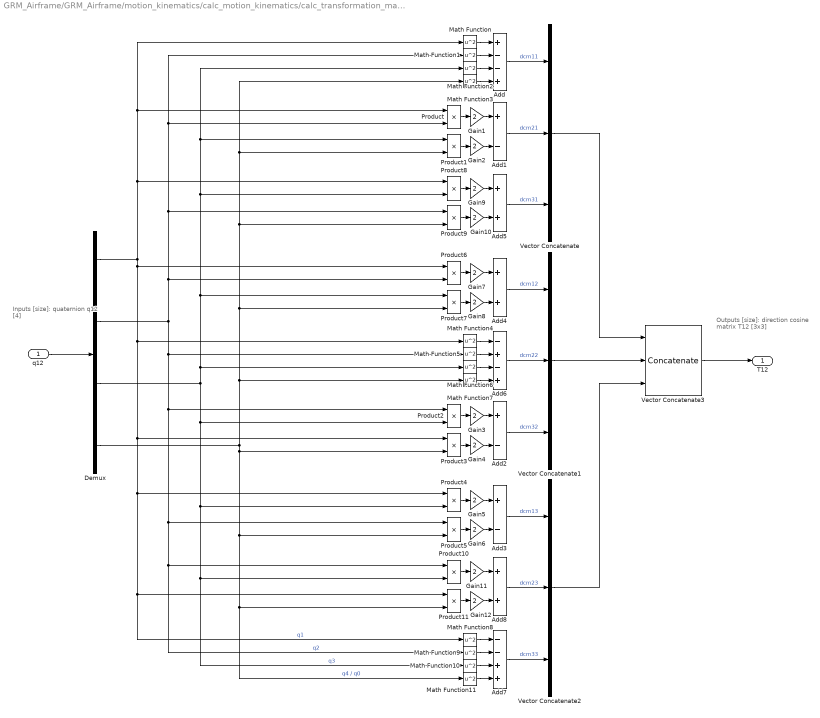
== system GRM_Airframe/GRM_Airframe/motion_kinematics/calc_motion_kinematics/calc_transformation_matrix/T12_from_q2 ==
  note: Outputs [size]:
      |
      | direction cosine matrix T12 [3x3]
  note: Inputs [size]:
      |
      | quaternion q12 [4]
  q12 : Inport  PortDimensions=4
  Add : Sum  Inputs=+--+
  Add1 : Sum  Inputs=+-
  Add2 : Sum  Inputs=+-
  Add3 : Sum  Inputs=+-
  Add4 : Sum
  Add5 : Sum
  Add6 : Sum  Inputs=-+-+
  Add7 : Sum  Inputs=--++
  Add8 : Sum
  Demux : Demux
  Gain{1..12} (12 alike) : Gain  Gain=2
  Math Function{,1..11} (12 alike) : Math  Operator=square  SaturateOnIntegerOverflow=on
  Product{,1..11} (12 alike) : Product
  Vector Concatenate : Concatenate  NumInputs=3
  Vector Concatenate1 : Concatenate  NumInputs=3
  Vector Concatenate2 : Concatenate  NumInputs=3
  Vector Concatenate3 : Concatenate  NumInputs=3  Mode=Multidimensional array  ConcatenateDimension=2
  T12 : Outport  PortDimensions=[3 3]
  wires:
  q12/1 -> Demux/1
  Demux/1 -> Product8/1, Product/1, Math Function/1, Product3/1, Product4/1, Product11/1, Math Function8/1, Math Function4/1, Product6/1  "q1"
  Demux/2 -> Product2/1, Product5/1, Product10/1, Math Function9/1, Math Function5/1, Product6/2, Product9/1, Product/2, Math Function1/1  "q2"
  Demux/3 -> Product2/2, Product4/2, Math Function10/1, Product10/2, Math Function6/1, Product7/1, Product8/2, Product1/1, Math Function2/1  "q3"
  Demux/4 -> Math Function7/1, Product7/2, Product9/2, Product1/2, Math Function3/1, Product5/2, Math Function11/1, Product11/2, Product3/2  "q4 / q0"
  Vector Concatenate3/1 -> T12/1
  Vector Concatenate/1 -> Vector Concatenate3/1
  Vector Concatenate2/1 -> Vector Concatenate3/3
  Vector Concatenate1/1 -> Vector Concatenate3/2
  Add/1 -> Vector Concatenate/1  "dcm11"
  Add1/1 -> Vector Concatenate/2  "dcm21"
  Add5/1 -> Vector Concatenate/3  "dcm31"
  Add4/1 -> Vector Concatenate1/1  "dcm12"
  Add6/1 -> Vector Concatenate1/2  "dcm22"
  Add2/1 -> Vector Concatenate1/3  "dcm32"
  Add3/1 -> Vector Concatenate2/1  "dcm13"
  Add8/1 -> Vector Concatenate2/2  "dcm23"
  Add7/1 -> Vector Concatenate2/3  "dcm33"
  Math Function/1 -> Add/1
  Math Function1/1 -> Add/2
  Math Function2/1 -> Add/3
  Math Function3/1 -> Add/4
  Product/1 -> Gain1/1
  Product1/1 -> Gain2/1
  Gain1/1 -> Add1/1
  Gain2/1 -> Add1/2
  Gain4/1 -> Add2/2
  Gain3/1 -> Add2/1
  Product3/1 -> Gain4/1
  Product2/1 -> Gain3/1
  Gain6/1 -> Add3/2
  Gain5/1 -> Add3/1
  Product5/1 -> Gain6/1
  Product4/1 -> Gain5/1
  Gain8/1 -> Add4/2
  Gain7/1 -> Add4/1
  Product7/1 -> Gain8/1
  Product6/1 -> Gain7/1
  Gain10/1 -> Add5/2
  Gain9/1 -> Add5/1
  Product9/1 -> Gain10/1
  Product8/1 -> Gain9/1
  Math Function6/1 -> Add6/3
  Math Function7/1 -> Add6/4
  Math Function5/1 -> Add6/2
  Math Function4/1 -> Add6/1
  Math Function10/1 -> Add7/3
  Math Function11/1 -> Add7/4
  Math Function9/1 -> Add7/2
  Math Function8/1 -> Add7/1
  Gain12/1 -> Add8/2
  Gain11/1 -> Add8/1
  Product11/1 -> Gain12/1
  Product10/1 -> Gain11/1

== system GRM_Airframe/GRM_Airframe/motion_kinematics/calc_motion_kinematics/calc_transformation_matrix/conjugate_quaternion ==
  note: Inputs [size]:
      |
      | q [4]
  note: Outputs [size]:
      |
      | q_conj [4]
  q : Inport
  Demux : Demux  Outputs=[3;1]
  Gain1 : Gain  Gain=-1
  Vector Concatenate : Concatenate
  q_conj : Outport
  wires:
  q/1 -> Demux/1
  Vector Concatenate/1 -> q_conj/1
  Demux/1 -> Gain1/1
  Gain1/1 -> Vector Concatenate/1
  Demux/2 -> Vector Concatenate/2

== system GRM_Airframe/GRM_Airframe/motion_kinematics/calc_motion_kinematics/calc_transformation_matrix/q31_from_q32_mul_q1 ==
  note: Inputs [size]:
      |
      | quaternion q32 [4]
      | quaternion q21 [4]
  note: Outputs [size]:
      |
      | quaternion q31 [4]
  q32 : Inport
  q21 : Inport  Port=2
  Add : Sum  Inputs=++++
  Constant : Constant
  Constant1 : Constant  Value=-1
  Demux1 : Demux
  Product{,1..4} (5 alike) : Product
  Product8 : Product  Multiplication=Matrix(*)
  Q_1 : Constant  Value=[0 0 0 1; 0 0 1 0; 0 -1 0 0; -1 0 0 0]
  Q_2 : Constant  Value=[0 0 -1 0; 0 0 0 1; 1 0 0 0; 0 -1 0 0]
  Q_3 : Constant  Value=[0 1 0 0; -1 0 0 0; 0 0 0 1; 0 0 -1 0]
  Q_4 : Constant  Value=[1 0 0 0; 0 1 0 0; 0 0 1 0; 0 0 0 1]
  Selector : Selector  IndexMode=Zero-based  InputPortWidth=4  IndexOptions=Index vector (dialog)  Indices=3  OutputSizes=1
  Switch : Switch
  normalize_quaternion : Subsystem
      mask help: normalize a quaternion
      mask Help:
      | Name:
      | 
      |     normalize_quaternion
      | 
      | Description:
      | 
      |     This block normalizes the quaternion q21. It should be used as a
      |     safety measure when computing quaternions.
      | 
      | Inputs  [size] [data type] [unit]:
      | 
      |     attitude quaternion q21  [4] [double] [-]
      | 
      | Outputs  [size] [data type] [unit]:
      | 
      |     normalized attitude quaternion q21  [4] [double] [-]
      mask Display: disp (' norm(q)')
  q31 : Outport
  wires:
  q21/1 -> Product8/2
  Demux1/1 -> Product/2  "q1"
  Demux1/2 -> Product1/2  "q2"
  Demux1/3 -> Product2/2  "q3"
  Demux1/4 -> Product3/2  "q4"
  Q_1/1 -> Product/1
  Q_2/1 -> Product1/1
  Q_3/1 -> Product2/1
  Q_4/1 -> Product3/1
  Product/1 -> Add/1
  Product1/1 -> Add/2
  Product2/1 -> Add/3
  Product3/1 -> Add/4
  Add/1 -> Product8/1  "Q(q32)"
  q32/1 -> Demux1/1
  Product8/1 -> normalize_quaternion/1(q)
  normalize_quaternion/1(q_normalized) -> Product4/1, Selector/1
  Selector/1 -> Switch/2
  Product4/1 -> q31/1
  Constant1/1 -> Switch/3
  Constant/1 -> Switch/1
  Switch/1 -> Product4/2

== system GRM_Airframe/GRM_Airframe/motion_kinematics/calc_motion_kinematics/calc_transformation_matrix/q31_from_q32_mul_q2 ==
  note: Inputs [size]:
      |
      | quaternion q32 [4]
      | quaternion q21 [4]
  note: Outputs [size]:
      |
      | quaternion q31 [4]
  q32 : Inport
  q21 : Inport  Port=2
  Add : Sum  Inputs=++++
  Constant : Constant
  Constant1 : Constant  Value=-1
  Demux1 : Demux
  Product{,1..4} (5 alike) : Product
  Product8 : Product  Multiplication=Matrix(*)
  Q_1 : Constant  Value=[0 0 0 1; 0 0 1 0; 0 -1 0 0; -1 0 0 0]
  Q_2 : Constant  Value=[0 0 -1 0; 0 0 0 1; 1 0 0 0; 0 -1 0 0]
  Q_3 : Constant  Value=[0 1 0 0; -1 0 0 0; 0 0 0 1; 0 0 -1 0]
  Q_4 : Constant  Value=[1 0 0 0; 0 1 0 0; 0 0 1 0; 0 0 0 1]
  Selector : Selector  IndexMode=Zero-based  InputPortWidth=4  IndexOptions=Index vector (dialog)  Indices=3  OutputSizes=1
  Switch : Switch
  normalize_quaternion : Subsystem
      mask help: normalize a quaternion
      mask Help:
      | Name:
      | 
      |     normalize_quaternion
      | 
      | Description:
      | 
      |     This block normalizes the quaternion q21. It should be used as a
      |     safety measure when computing quaternions.
      | 
      | Inputs  [size] [data type] [unit]:
      | 
      |     attitude quaternion q21  [4] [double] [-]
      | 
      | Outputs  [size] [data type] [unit]:
      | 
      |     normalized attitude quaternion q21  [4] [double] [-]
      mask Display: disp (' norm(q)')
  q31 : Outport
  wires:
  q21/1 -> Product8/2
  Demux1/1 -> Product/2  "q1"
  Demux1/2 -> Product1/2  "q2"
  Demux1/3 -> Product2/2  "q3"
  Demux1/4 -> Product3/2  "q4"
  Q_1/1 -> Product/1
  Q_2/1 -> Product1/1
  Q_3/1 -> Product2/1
  Q_4/1 -> Product3/1
  Product/1 -> Add/1
  Product1/1 -> Add/2
  Product2/1 -> Add/3
  Product3/1 -> Add/4
  Add/1 -> Product8/1  "Q(q32)"
  q32/1 -> Demux1/1
  Product8/1 -> normalize_quaternion/1(q)
  normalize_quaternion/1(q_normalized) -> Product4/1, Selector/1
  Selector/1 -> Switch/2
  Product4/1 -> q31/1
  Constant1/1 -> Switch/3
  Constant/1 -> Switch/1
  Switch/1 -> Product4/2

== system GRM_Airframe/GRM_Airframe/motion_kinematics/calc_motion_kinematics/calc_transformation_matrix/q31_from_q32_mul_q21 ==
  note: Inputs [size]:
      |
      | quaternion q32 [4]
      | quaternion q21 [4]
  note: Outputs [size]:
      |
      | quaternion q31 [4]
  q32 : Inport
  q21 : Inport  Port=2
  Add : Sum  Inputs=++++
  Constant : Constant
  Constant1 : Constant  Value=-1
  Demux1 : Demux
  Product{,1..4} (5 alike) : Product
  Product8 : Product  Multiplication=Matrix(*)
  Q_1 : Constant  Value=[0 0 0 1; 0 0 1 0; 0 -1 0 0; -1 0 0 0]
  Q_2 : Constant  Value=[0 0 -1 0; 0 0 0 1; 1 0 0 0; 0 -1 0 0]
  Q_3 : Constant  Value=[0 1 0 0; -1 0 0 0; 0 0 0 1; 0 0 -1 0]
  Q_4 : Constant  Value=[1 0 0 0; 0 1 0 0; 0 0 1 0; 0 0 0 1]
  Selector : Selector  IndexMode=Zero-based  InputPortWidth=4  IndexOptions=Index vector (dialog)  Indices=3  OutputSizes=1
  Switch : Switch
  normalize_quaternion : Subsystem
      mask help: normalize a quaternion
      mask Help:
      | Name:
      | 
      |     normalize_quaternion
      | 
      | Description:
      | 
      |     This block normalizes the quaternion q21. It should be used as a
      |     safety measure when computing quaternions.
      | 
      | Inputs  [size] [data type] [unit]:
      | 
      |     attitude quaternion q21  [4] [double] [-]
      | 
      | Outputs  [size] [data type] [unit]:
      | 
      |     normalized attitude quaternion q21  [4] [double] [-]
      mask Display: disp (' norm(q)')
  q31 : Outport
  wires:
  q21/1 -> Product8/2
  Demux1/1 -> Product/2  "q1"
  Demux1/2 -> Product1/2  "q2"
  Demux1/3 -> Product2/2  "q3"
  Demux1/4 -> Product3/2  "q4"
  Q_1/1 -> Product/1
  Q_2/1 -> Product1/1
  Q_3/1 -> Product2/1
  Q_4/1 -> Product3/1
  Product/1 -> Add/1
  Product1/1 -> Add/2
  Product2/1 -> Add/3
  Product3/1 -> Add/4
  Add/1 -> Product8/1  "Q(q32)"
  q32/1 -> Demux1/1
  Product8/1 -> normalize_quaternion/1(q)
  normalize_quaternion/1(q_normalized) -> Product4/1, Selector/1
  Selector/1 -> Switch/2
  Product4/1 -> q31/1
  Constant1/1 -> Switch/3
  Constant/1 -> Switch/1
  Switch/1 -> Product4/2
